simulink model "motomatic_pend_OL"  (R2020b)
settings: Solver=VariableStepAuto  StartTime=0.0  StopTime=2  FixedStep=1e-6  RelTol=1e-7
values from neighbouring files (symbols this model uses):
  Vin = position.Channel2_V_    [findKp.m]
undefined symbols (not defined in the file or in its folder): Ka, Kp, Kt, N, physParam, th_init
settings Model: Creator=Bradley Kwan  LastModifiedBy=Bradley Kwan

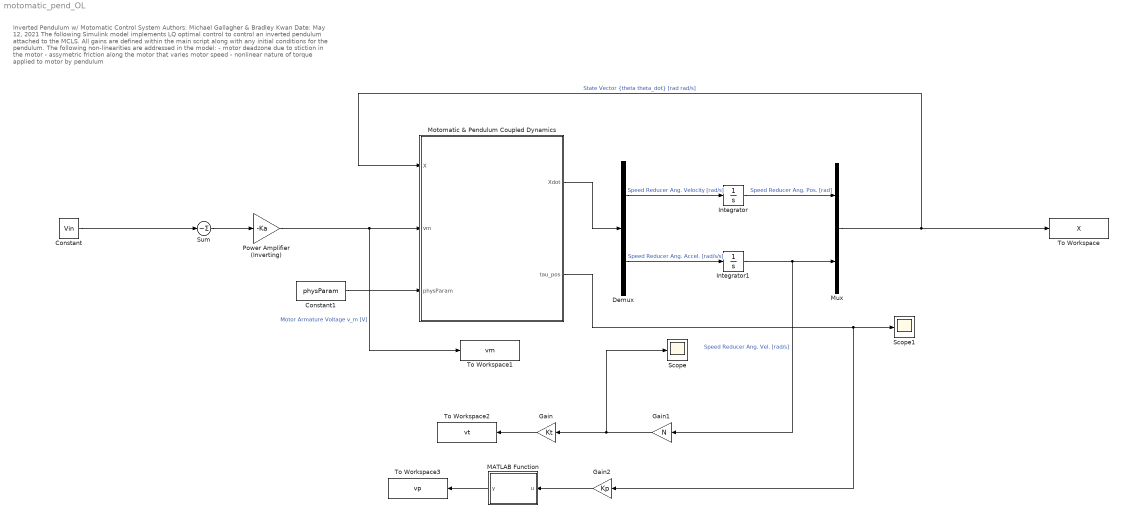
== system motomatic_pend_OL ==
  note: Inverted Pendulum w/ Motomatic Control System
      | Authors: Michael Gallagher & Bradley Kwan
      | Date: May 12, 2021
      |
      | The following Simulink model implements LQ optimal control to control an inverted pendulum attached to the MCLS. All gains are defined within the main script along with any initial conditions for the pendulum. The following non-linearities are addressed in the model:
      |
      | - motor deadzone due to stiction in the motor
      | - assymetric friction along the motor that varies motor speed
      | - nonlinear nature of torque applied to motor by pendulum
  Constant : Constant  Value=Vin
  Constant1 : Constant  Value=physParam
  Demux : Demux  Outputs=2
  Gain : Gain  Gain=Kt
  Gain1 : Gain  Gain=N
  Gain2 : Gain  Gain=Kp
  Integrator : Integrator  InitialCondition=th_init
  Integrator1 : Integrator
  MATLAB Function : MATLAB Function  TreatAsAtomicUnit=on
  Motomatic & Pendulum Coupled Dynamics : MATLAB Function  TreatAsAtomicUnit=on
  Mux : Mux  Inputs=2
  Power Amplifier (Inverting) : Gain  Gain=-Ka
  Scope : Scope
  Scope1 : Scope
  Sum : Sum  Inputs=-
  To Workspace : ToWorkspace  VariableName=X  SampleTime=-1
  To Workspace1 : ToWorkspace  VariableName=vm  SampleTime=-1
  To Workspace2 : ToWorkspace  VariableName=vt  SampleTime=-1
      settings: Save2DSignal=2-D array (concatenate along first dimension)
  To Workspace3 : ToWorkspace  VariableName=vp  SampleTime=-1
      settings: Save2DSignal=2-D array (concatenate along first dimension)
  wires:
  Constant1/1 -> Motomatic & Pendulum Coupled Dynamics/3(physParam)
  Motomatic & Pendulum Coupled Dynamics/1(Xdot) -> Demux/1
  Demux/1 -> Integrator/1  "Speed Reducer Ang. Velocity [rad/s]"
  Demux/2 -> Integrator1/1  "Speed Reducer Ang. Accel. [rad/s/s]"
  Integrator/1 -> Mux/1  "Speed Reducer Ang. Pos. [rad]"
  Integrator1/1 -> Gain1/1, Mux/2  "Speed Reducer Ang. Vel. [rad/s]"
  Mux/1 -> To Workspace/1, Motomatic & Pendulum Coupled Dynamics/1(X)  "State Vector {theta theta_dot} [rad rad/s]"
  Power Amplifier (Inverting)/1 -> To Workspace1/1, Motomatic & Pendulum Coupled Dynamics/2(vm)  "Motor Armature Voltage v_m [V]"
  Constant/1 -> Sum/1
  Sum/1 -> Power Amplifier (Inverting)/1
  Gain1/1 -> Gain/1, Scope/1
  Gain/1 -> To Workspace2/1
  Motomatic & Pendulum Coupled Dynamics/2(tau_pos) -> Gain2/1, Scope1/1
  Gain2/1 -> MATLAB Function/1(u)
  MATLAB Function/1(y) -> To Workspace3/1

== matlab function motomatic_pend_OL/MATLAB Function ==
  data: u input; y output
function y = fcn(u)

if u>0
   y = u-18.5;
else
    y = 0;
end

== matlab function motomatic_pend_OL/Motomatic & Pendulum Coupled Dynamics ==
  data: X input; Xdot output; vm input; physParam input; tau_pos output
function [Xdot,tau_pos] = motor_dynamics(X,vm, physParam)

% First define the physical parameters of the pendulum model
M = physParam(1);      % bob mass [kg]
L = physParam(2);      % pendulum length [m]
g = physParam(3);      % gravitational acceleration [m/s/s]
vmo = physParam(4);    % Voltage necessary to hold pendulum at 90 degrees [v]
N = physParam(5);      % speed reducer factor
Km = physParam(6);

% Based on the physical parameters of the model, find the polar moments of
% inertia of the motor and pendulum
J_p = M*L^2;                    % Polar moment inertia of pendulum [kg*m^2]
J_m = M*g*L/vmo*(.2740/19.763); % Polar moment inertia of motor [kg*m^2]

Xdot = [NaN NaN];
tau_pos = X(1);
while tau_pos > 2*pi
   tau_pos = tau_pos-2*pi;
end
% First the function tests to see if the motor will overcome stiction
if abs(vm) < .832 && X(2) == 0 
    Xdot = [0 0];
else
    tau_m = .274;
    if tau_pos < pi/4
        tau_m = .240;
    elseif tau_pos > pi/2 && tau_pos < 3*pi/2
        tau_m = .290;
    end
    Xdot(1) = X(2);
    Xdot(2) = -1/tau_m*X(2) + ...
              Km/tau_m/N*vm;
end
